simulink library "Storage_Type_5_CONF"  (Simulink 8.2)
settings: Solver=ode45  StartTime=0.0  StopTime=10.0  RelTol=1e-3
libraries: carnot x2
settings Model: Creator=lena.frank  LastModifiedBy=drhf

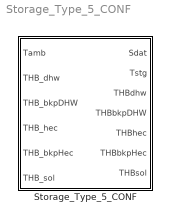
== system Storage_Type_5_CONF ==
  Storage_Type_5_CONF : Subsystem  mask(Combi-storage for hot water production and heating){parameterfile=Default_Storage, tini=[10:5:55]}
      mask prompts: parameterfile "Storage parameter set"; tini "initial temperature (vector or scalar) in °C"
      mask help: Predefinded combi-storage for hot water production and heating configurated for parallel buffer operation of the backup heater.
      mask init:
      | % callback to set parameters of model
      | CarnotCallbacks_StorageConf(5,parameterfile);
      mask Help: web(fullfile(path_carnot('help'),'Storage_Type_N.html'),'-helpbrowser')
      mask TypeOptions parameterfile: Default_Storage
      mask Display:
      | % user defined picture file
      | picfile = fullfile(path_carnot('intlibsl'), ...
      |         'Storage','Thermal','Storage_Type_5_CONF','parameter_set', ...
      |         'Storage_Type_5_CONF.jpg');
      | 
      | % show public picture
      | plot([36,36,40,50,54,54,50,40,36]/100,[90,50,45,45,50,90,93,93,90]/100, ...
      |     [36,51,40,51,36]/100,[50,50,68,85,85]/100,[36,51,44,51,36]/100, ...
      |     [54,54,56,58,58]/100)
      | 
      | % show internal picture if defined
      | if  ~BlockIsInCarnotLibrary       % if not located in library
      |     if exist(picfile)
      |         image(imread(picfile), [0.3, 0, 0.45, 1])
      |         set_param(gcb, 'BackgroundColor', 'White')
      |     end
      | end

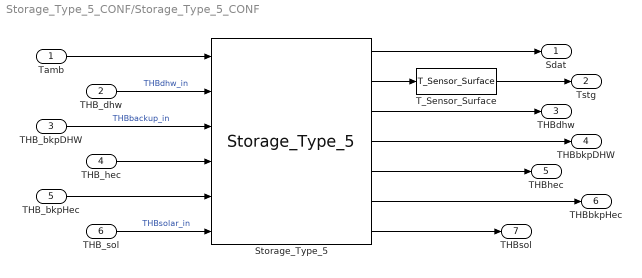
== system Storage_Type_5_CONF/Storage_Type_5_CONF ==
  Tamb : Inport
  THB_dhw : Inport  Port=2
  THB_bkpDHW : Inport  Port=3
  THB_hec : Inport  Port=4
  THB_bkpHec : Inport  Port=5
  THB_sol : Inport  Port=6
  Storage_Type_5 : carnot/Storage/Thermal/Storage_Type_5  uloss=0.74  ubot=1.37  utop=0.74  cond=0.62  t0=tini  volume=0.75  dia=0.79  pos=standing cylinder  nconnect=5  nodes=50  mpoints=50
  T_Sensor_Surface : carnot/Control/T_Sensor_Surface  pos=[0.1 0.5 0.7]  tdel=10  t0=tini(1)
  Sdat : Outport
  Tstg : Outport  Port=2
  THBdhw : Outport  Port=3
  THBbkpDHW : Outport  Port=4
  THBhec : Outport  Port=5
  THBbkpHec : Outport  Port=6
  THBsol : Outport  Port=7
  wires:
  THB_hec/1 -> Storage_Type_5/4
  Storage_Type_5/6 -> THBbkpHec/1
  Storage_Type_5/5 -> THBhec/1
  Storage_Type_5/2 -> T_Sensor_Surface/1
  Storage_Type_5/1 -> Sdat/1
  THB_sol/1 -> Storage_Type_5/6  "THBsolar_in"
  THB_bkpDHW/1 -> Storage_Type_5/3  "THBbackup_in"
  THB_dhw/1 -> Storage_Type_5/2  "THBdhw_in"
  Tamb/1 -> Storage_Type_5/1
  Storage_Type_5/3 -> THBdhw/1
  Storage_Type_5/4 -> THBbkpDHW/1
  Storage_Type_5/7 -> THBsol/1
  THB_bkpHec/1 -> Storage_Type_5/5
  T_Sensor_Surface/1 -> Tstg/1
